simulink model "MassSpringDamperModel"  (R2021a)
settings: Solver=VariableStepAuto  StartTime=0.0  StopTime=20  RelTol=1e-3  AbsTol=1e-6
PreLoadFcn:
  | prms.mass = 2; % kg
  | prms.damping = 3; % N/m/s
  | prms.stiffness = 128; % N/m
  | prms.restitution = 0.9;
  | 
  | prms.pos.min = -0.2; % m
  | prms.pos.ini =  0.5; % m
  | prms.pos.max =  inf; % m
  | 
  | prms.vel.min = -realmax; % m/s, can't use inf, bug. grr.
  | prms.vel.ini =  0.0; % m/s
  | prms.vel.max =  realmax; % m/s, can't use inf, bug. grr.
model workspace (MAT data in the model file):
  b = 3
  k = 128
  m = 2
  x0 = 0.5
Description:
  | The van der Pol Equation
  | 
  | This is a simulation of a nonlinear second order system.
settings Model: SimulationMode=rapid-accelerator  ExtModeAutoUpdateStatusClock=off  OrderedModelArguments=off  Creator=The MathWorks, Inc.  LastModifiedBy=ewlee
settings SolverCC: AutoScaleAbsTol=off  AlgebraicLoopSolver=TrustRegion
settings DataIOCC: ExternalInput=[]  InitialState=[]  SaveFormat=StructureWithTime  SignalLogging=off  DSMLogging=off  SaveTime=off  TimeSaveName=t  OutputSaveName=y
settings OptimizationCC: BlockReduction=off  BooleanDataType=off  InitFltsAndDblsToZero=on  LifeSpan=inf  BufferReusableBoundary=off
settings DebuggingCC: SaveWithParameterizedLinksMsg=none  SignalResolutionControl=TryResolveAllWithWarning  MultiTaskDSMMsg=warning  MultiTaskCondExecSysMsg=none  FcnCallInpInsideContextMsg=warning  BusObjectLabelMismatch=none  PregeneratedLibrarySubsystemCodeDiagnostic=none  SFUnexpectedBacktrackingDiag=warning  SFNoUnconditionalDefaultTransitionDiag=warning  SFExecutionAtInitializationDiag=none  SFMachineParentedDataDiag=warning  ArithmeticOperatorsInVariantConditions=warning
settings HardwareCC: ProdBitPerPointer=32  ProdBitPerSizeT=32  ProdBitPerPtrDiffT=32  ProdLargestAtomicFloat=None  ProdIntDivRoundTo=Undefined  ProdEndianess=Unspecified  ProdWordSize=32  ProdHWDeviceType=32-bit Generic  TargetUnknown=on
settings ModelReferenceCC: PropagateSignalLabelsOutOfModel=off
settings SFSimCC: SimUseLocalCustomCode=off
settings RTWCC: Description=Generic Real-Time Target  RTWUseLocalCustomCode=off
settings CodeAppCC: StateflowObjectComments=on
settings GRTTargetCC: TargetFcnLib=ansi_tfl_tmw.mat  TargetLangStandard=C89/C90 (ANSI)  CombineOutputUpdateFcns=off  GRTInterface=on
settings ConfigComp: CovMetricSettings=dw  CovSaveCumulativeToWorkspaceVar=on  CovSaveSingleToWorkspaceVar=on  CovExternalEMLEnable=off

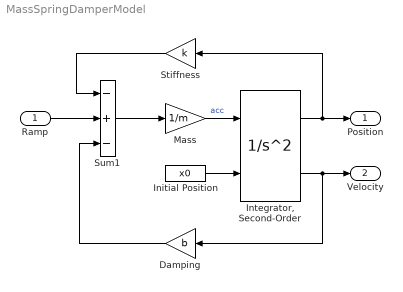
== system MassSpringDamperModel ==
  Ramp : Inport
  Damping : Gain  Gain=b
  Initial Position : Constant  Value=x0
  "Integrator, Second-Order" : SecondOrderIntegrator  ICSourceX=external  StateNameX='pos'  StateNameDXDT='vel'  ReinitDXDTwhenXreachesSaturation=on
  Mass : Gain  Gain=1/m
  Stiffness : Gain  Gain=k
  Sum1 : Sum  Inputs=-+-
  Position : Outport  VectorParamsAs1DForOutWhenUnconnected=off
  Velocity : Outport  Port=2  VectorParamsAs1DForOutWhenUnconnected=off
  wires:
  Sum1/1 -> Mass/1
  Mass/1 -> "Integrator, Second-Order"/1  "acc"
  Ramp/1 -> Sum1/2
  "Integrator, Second-Order"/1 -> Stiffness/1, Position/1
  Stiffness/1 -> Sum1/1
  "Integrator, Second-Order"/2 -> Damping/1, Velocity/1
  Initial Position/1 -> "Integrator, Second-Order"/2
  Damping/1 -> Sum1/3
